simulink model "EX4zadanie1"  (R2023b)
settings: Solver=FixedStepDiscrete  StartTime=0.0  StopTime=0.0  RelTol=1e-3
libraries: CPOiS_SourcesSinks x8, CPOiS_DataManipulation_IntroduceNoise x2, CPOiS_LinearTransforms x2, CPOiS_DataManipulation_DataTypeConversion x2
settings Model: Creator=kkarkosz  LastModifiedBy=alyskawa

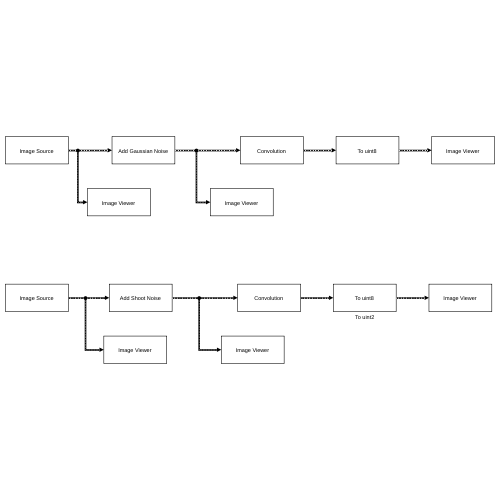
[thumbnail: Simulink's stored preview of the top-level diagram]
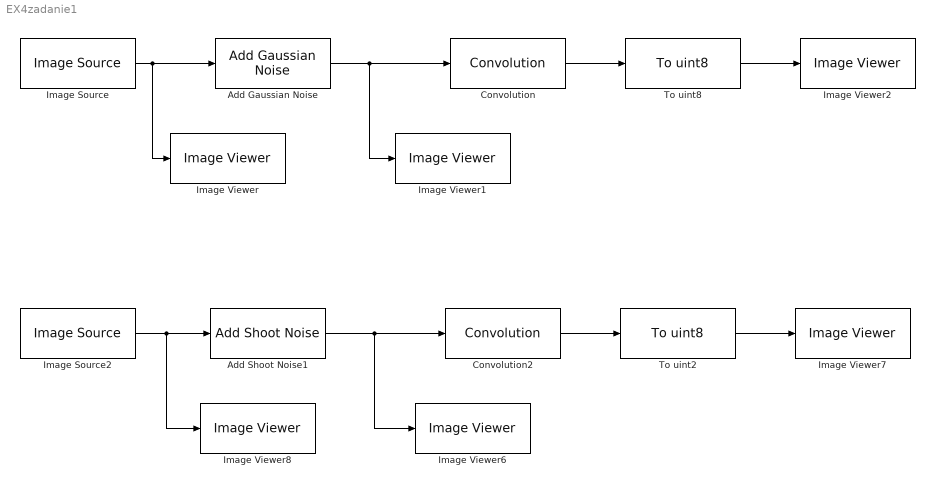
== system EX4zadanie1 ==
  Add Gaussian Noise : CPOiS_DataManipulation_IntroduceNoise/Add Gaussian Noise  Mean=8.0  Variance=1
      settings: SourceProductName=CPOiS - Digital image and signal processing
  Add Shoot Noise1 : CPOiS_DataManipulation_IntroduceNoise/Add Shoot Noise  Density=15
      settings: SourceProductName=CPOiS - Digital image and signal processing
  Convolution : CPOiS_LinearTransforms/Convolution  ConvolutionMatrix=1/(sum(sum([1; 2; 1] * [1; 2; 1]'))) * [1; 2; 1] * [1; 2; 1]'
      settings: SourceProductName=CPOiS - Digital image and signal processing
  Convolution2 : CPOiS_LinearTransforms/Convolution  ConvolutionMatrix=1/(sum(sum([1; 2; 1] * [1; 2; 1]'))) * [1; 2; 1] * [1; 2; 1]'
      settings: SourceProductName=CPOiS - Digital image and signal processing
  Image Source : CPOiS_SourcesSinks/Image Source  FileSelection=gull.png
      settings: SourceProductName=CPOiS - Digital image and signal processing
  Image Source2 : CPOiS_SourcesSinks/Image Source  FileSelection=gull.png
      settings: SourceProductName=CPOiS - Digital image and signal processing
  Image Viewer{,1..2,6..8} (6 alike) : CPOiS_SourcesSinks/Image Viewer
      settings: SourceProductName=CPOiS - Digital image and signal processing
  To uint2 : CPOiS_DataManipulation_DataTypeConversion/To uint8
      settings: SourceProductName=CPOiS - Digital image and signal processing
  To uint8 : CPOiS_DataManipulation_DataTypeConversion/To uint8
      settings: SourceProductName=CPOiS - Digital image and signal processing
  wires:
  Image Source/1 -> Add Gaussian Noise/1, Image Viewer/1
  Add Gaussian Noise/1 -> Image Viewer1/1, Convolution/1
  Convolution/1 -> To uint8/1
  To uint8/1 -> Image Viewer2/1
  To uint2/1 -> Image Viewer7/1
  Convolution2/1 -> To uint2/1
  Image Source2/1 -> Image Viewer8/1, Add Shoot Noise1/1
  Add Shoot Noise1/1 -> Image Viewer6/1, Convolution2/1
